simulink model "Alt_Control"  (R2015a)
settings: Solver=ode2  StartTime=0.0  StopTime=10.0  FixedStep=0.01  RelTol=1e-3
InitFcn:
  | Parameters
values from neighbouring files (symbols this model uses):
  KaD = 5.4    [Parameters.m]
  KaI = 3.6    [Parameters.m]
  KaN = 38    [Parameters.m]
  KaP = 8.0    (= 8)    [Parameters.m]
  Kba = sqrt(KaD/KaI)    [Parameters.m]
  sata = 5    [Parameters.m]
libraries: simulink x1
settings Model: Creator=pela  LastModifiedBy=Mattia
settings HardwareCC: ProdLargestAtomicInteger=Long  ProdLargestAtomicFloat=Double  ProdEndianess=LittleEndian  ProdHWDeviceType=ARM Compatible->ARM Cortex
settings RTWCC: GenCodeOnly=on  GenerateReport=on  Toolchain=Microsoft Visual C++ 2013 v12.0 | nmake (64-bit Windows)  BuildConfiguration=Faster Runs  LaunchReport=on  TargetLang=C++
settings GRTTargetCC: MatFileLogging=off  MultiInstanceERTCode=on  CodeInterfacePackaging=C++ class  SupportNonFinite=off

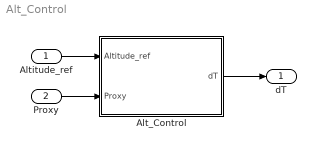
== system Alt_Control ==
  Altitude_ref : Inport
  Proxy : Inport  Port=2
  Alt_Control : Subsystem
  dT : Outport
  wires:
  Altitude_ref/1 -> Alt_Control/1(Altitude_ref)
  Proxy/1 -> Alt_Control/2(Proxy)
  Alt_Control/1(dT) -> dT/1

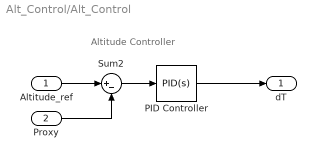
== system Alt_Control/Alt_Control ==
  note: Altitude Controller
  Altitude_ref : Inport
  Proxy : Inport  Port=2
  PID Controller : simulink/Continuous/PID Controller  Controller=PID  TimeDomain=Continuous-time  SampleTime=-1  IntegratorMethod=Forward Euler  FilterMethod=Trapezoidal  Form=Parallel  UseFilter=on  ControllerParametersSource=internal  P=KaP  I=KaI  D=KaD  N=KaN  InitialConditionSource=internal  InitialConditionForIntegrator=0  InitialConditionForFilter=0  ExternalReset=none  LimitOutput=on  UpperSaturationLimit=sata  LowerSaturationLimit=-sata  LinearizeAsGain=on  AntiWindupMode=back-calculation  Kb=Kba  TrackingMode=off  Kt=1  PParamMin=[]  PParamMax=[]  IParamMin=[]  IParamMax=[]  DParamMin=[]  DParamMax=[]  NParamMin=[]  NParamMax=[]  KbParamMin=[]  KbParamMax=[]  KtParamMin=[]  KtParamMax=[]  POutMin=[]  POutMax=[]  IOutMin=[]  IOutMax=[]  DOutMin=[]  DOutMax=[]  NOutMin=[]  NOutMax=[]  KbOutMin=[]  KbOutMax=[]  KtOutMin=[]  KtOutMax=[]  IntegratorOutMin=[]  IntegratorOutMax=[]  FilterOutMin=[]  FilterOutMax=[]  SumOutMin=[]  SumOutMax=[]  SumI1OutMin=[]  SumI1OutMax=[]  SumI2OutMin=[]  SumI2OutMax=[]  SumI3OutMin=[]  SumI3OutMax=[]  SumDOutMin=[]  SumDOutMax=[]  SaturationOutMin=[]  SaturationOutMax=[]  IntegratorContinuousStateAttributes=''  IntegratorStateMustResolveToSignalObject=off  IntegratorRTWStateStorageClass=Auto  FilterContinuousStateAttributes=''  FilterStateMustResolveToSignalObject=off  FilterRTWStateStorageClass=Auto  DifferentiatorICPrevScaledInput=0  DifferentiatorOutMin=[]  DifferentiatorOutMax=[]
  Sum2 : Sum  Inputs=|+-
  dT : Outport
  wires:
  Sum2/1 -> PID Controller/1
  Altitude_ref/1 -> Sum2/1
  Proxy/1 -> Sum2/2
  PID Controller/1 -> dT/1
